simulink model "F1_Telemetry_Universal"  (R2025a)
settings: Solver=FixedStepDiscrete  StartTime=0.0  StopTime=10.0  FixedStep=0.1  RelTol=1e-3
settings Model: Creator=sunda  LastModifiedBy=sunda

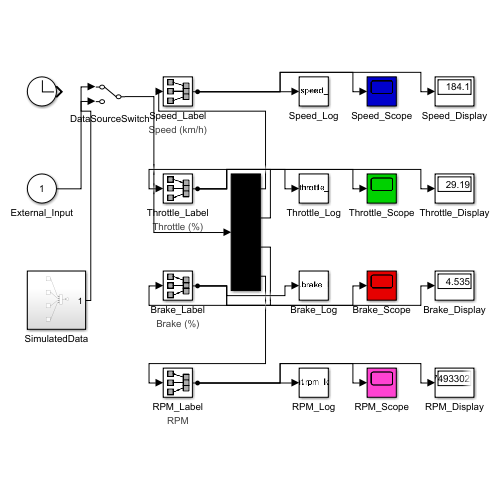
[thumbnail: Simulink's stored preview of the top-level diagram]
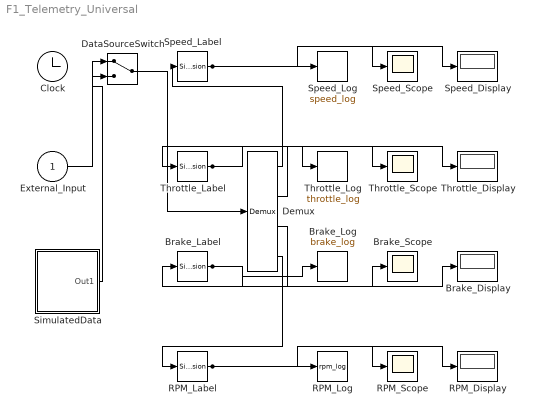
== system F1_Telemetry_Universal ==
  External_Input : Inport
  Brake_Display : Display
  Brake_Label : SignalConversion  OverrideOpt=off
      settings: AttributesFormatString=Brake (%)
  Brake_Log : ToWorkspace  VariableName=brake_log  SampleTime=-1
  Brake_Scope : Scope
      settings: ActiveDisplayYMinimum=-6.2476176155540069  ActiveDisplayYMaximum=56.249735290617117
  Clock : Clock
  DataSourceSwitch : ManualSwitch
  Demux : Demux
  RPM_Display : Display
      settings: Format=decimal (Stored Integer)
  RPM_Label : SignalConversion  OverrideOpt=off
      settings: AttributesFormatString=RPM
  RPM_Log : ToWorkspace  VariableName=rpm_log  SampleTime=-1
  RPM_Scope : Scope
      settings: ActiveDisplayYMinimum=6376.5656333724664  ActiveDisplayYMaximum=12610.909299647803
  SimulatedData : Subsystem
  Speed_Display : Display
  Speed_Label : SignalConversion  OverrideOpt=off
      settings: AttributesFormatString=Speed (km/h)
  Speed_Log : ToWorkspace  VariableName=speed_log  SampleTime=-1
  Speed_Scope : Scope
      settings: ActiveDisplayYMinimum=89.481612689901311  ActiveDisplayYMaximum=194.66548579088823
  Throttle_Display : Display
  Throttle_Label : SignalConversion  OverrideOpt=off
      settings: AttributesFormatString=Throttle (%)
  Throttle_Log : ToWorkspace  VariableName=throttle_log  SampleTime=-1
  Throttle_Scope : Scope
      settings: ActiveDisplayYMinimum=20.341740444223273  ActiveDisplayYMaximum=108.85091772841963
  wires:
  SimulatedData/1(Out1) -> DataSourceSwitch/1
  External_Input/1 -> DataSourceSwitch/2
  DataSourceSwitch/1 -> Demux/1
  Demux/1 -> Speed_Label/1
  Speed_Label/1 -> Speed_Log/1, Speed_Scope/1, Speed_Display/1
  Demux/2 -> Throttle_Label/1
  Throttle_Label/1 -> Throttle_Log/1, Throttle_Scope/1, Throttle_Display/1
  Demux/3 -> Brake_Label/1
  Brake_Label/1 -> Brake_Log/1, Brake_Scope/1, Brake_Display/1
  Demux/4 -> RPM_Label/1
  RPM_Label/1 -> RPM_Log/1, RPM_Scope/1, RPM_Display/1

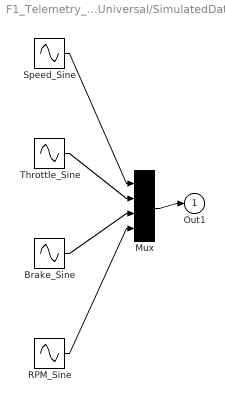
== system F1_Telemetry_Universal/SimulatedData ==
  Brake_Sine : Sin  Amplitude=50  Bias=50  Frequency=0.2  Phase=pi  SampleTime=0.1
  Mux : Mux
  RPM_Sine : Sin  Amplitude=5000  Bias=7000  Frequency=0.15  SampleTime=0.1
  Speed_Sine : Sin  Amplitude=100  Bias=100  Frequency=0.1  SampleTime=0.1
  Throttle_Sine : Sin  Amplitude=50  Bias=50  Frequency=0.2  Phase=pi/2  SampleTime=0.1
  Out1 : Outport
  wires:
  Speed_Sine/1 -> Mux/1
  Throttle_Sine/1 -> Mux/2
  Brake_Sine/1 -> Mux/3
  RPM_Sine/1 -> Mux/4
  Mux/1 -> Out1/1
